simulink library "commcnvintrlv2"  (Simulink 5.0)
libraries: commcnvintrlv2 x4, dspsigattribs x4, commblksprivate x2, commblkintrlv2 x2, simulink x2, dspsigops x1
settings Model: RequirementInfo=9  Creator=mikem  LastModifiedBy=mmclerno  TargetHWChar=2  TargetHWWordLengths=8,16,32,32

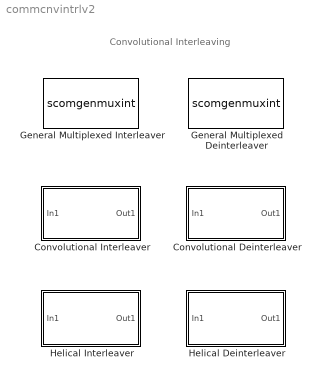
== system commcnvintrlv2 ==
  note: Convolutional Interleaving
  Convolutional Deinterleaver : Subsystem  mask(Convolutional Deinterleaver){N=6, B=2, ic=0}
      mask prompts: N "Rows of shift registers:"; B "Register length step:"; ic "Initial conditions:"
      mask help: A convolutional deinterleaver consists of N shift registers. The ith register has delay (N-i)*B where B is a specified register length step. With each new input symbol, a commutator switches to a new register and the new symbol is shifted in while the oldest symbol in that register is shifted out. When the commutator reaches the Nth register, upon the next new input, it returns to the first register.
      mask Help: helpview(commbhelp)
      mask Display: disp('Convolutional\nDeinterleaver');
  Convolutional Interleaver : Subsystem  mask(Convolutional Interleaver){N=6, B=2, ic=0}
      mask prompts: N "Rows of shift registers:"; B "Register length step:"; ic "Initial conditions:"
      mask help: A convolutional interleaver consists of N shift registers. The ith register has delay (i-1)*B where B is a specified register length step. With each new input symbol, a commutator switches to a new register and the new symbol is shifted in while the oldest symbol in that register is shifted out. When the commutator reaches the Nth register, upon the next new input, it returns to the first register.
      mask Help: helpview(commbhelp)
      mask Display: disp('Convolutional\nInterleaver');
  General Multiplexed Deinterleaver : S-Function  FunctionName=scomgenmuxint  Parameters=delayinverse, real(ic), imag(ic)  mask(General Multiplexed Deinterleaver){delay=[2 0 1 3 10], ic=0}
      mask prompts: delay "Interleaver delay (samples):"; ic "Initial conditions:"
      mask help:
      | A general multiplexed deinterleaver consists of N registers.  With each new input symbol, a commutator switches to a new register and the new symbol is shifted in while the oldest symbol in that register is shifted out.  When the commutator reaches the Nth register, upon the next new input, it returns to the first register.
      |
      | The multiplexed deinterleaver associated with a general multiplexed interleaver has the same number of registers as the interleaver.  The delay in a particular deinterleaver register depends on the largest interleaver delay minus the interleaver delay for the given register.
      mask init:
      | delayinverse=max(delay)-delay;
      mask Help: helpview(commbhelp)
      mask Display: disp('General\nMultiplexed\nDeinterleaver');
  General Multiplexed Interleaver : S-Function  FunctionName=scomgenmuxint  Parameters=delay, real(ic), imag(ic)  mask(General Multiplexed Interleaver){delay=[2 0 1 3 10], ic=0}
      mask prompts: delay "Interleaver delay (samples):"; ic "Initial conditions:"
      mask help: A general multiplexed interleaver consists of N registers, each with a specified delay. With each new input symbol, a commutator switches to a new register and the new symbol is shifted in while the oldest symbol in that register is shifted out. When the commutator reaches the Nth register, upon the next new input, it returns to the first register.
      mask Help: helpview(commbhelp)
      mask Display: disp('General\nMultiplexed\nInterleaver');
  Helical Deinterleaver : Subsystem  mask(Helical Deinterleaver){C=6, N=4, s=1, ic=0}
      mask prompts: C "Number of columns in helical array:"; N "Group size:"; s "Helical array step size:"; ic "Initial condition:"
      mask help:
      | Restore the ordering of symbols input to a matching helical interleaver.  The operation of a helical deinterleaver is defined by a helical array with C columns.  The input to the helical deinterleaver must have width C*N.  Received symbols are entered row-by-row into the helical array.  The block processes the symbols in the helical array in groups of size N and assigns an index k to each group, beginning with k=1 at the start of the simulation.  After a delay, the kth output group is read sequentially down column k mod C of the helical array and beginning in row 1+(k-1)*s, where s is the helical array step size.
      |
      | The helical array step size must be a nonnegative integer and the initial condition must be a scalar.
      mask init:
      | if s<0
      |     error('The helical array step size must be a nonnegative integer.');
      | end
      | 
      | if length(ic)~=1
      |    error('The initial condition must be a scalar.');
      | end
      | 
      | if(C<=0)
      |    error('The number of columns in helical array must be a nonnegative integer.');
      | end
      | 
      | if(N<=0)
      |    error('The group size must be a nonnegative integer.');
      | end
      mask Help: helpview(commbhelp)
      mask Display: disp('Helical\nDeinterleaver');
  Helical Interleaver : Subsystem  mask(Helical Interleaver){C=6, N=4, s=1, ic=0}
      mask prompts: C "Number of columns in helical array:"; N "Group size:"; s "Helical array step size:"; ic "Initial condition:"
      mask help:
      | Permute input vector using a helical array with C columns.  The input to the helical interleaver must have width C*N.  The block processes the input in groups of size N and assigns an index to each group, beginning with k=1 at the start of the simulation.  The kth group of N symbols is entered sequentially down column k mod C of the helical array and beginning in row 1+(k-1)*s, where s is the helical array step size.  The helical interleaver output is then read row-by-row from the helical array.
      |
      | The helical array step size must be a nonnegative integer and the initial condition must be a scalar.
      mask init:
      | if s<0
      |     error('The helical array step size must be a nonnegative integer.');
      | end
      | 
      | if length(ic)~=1
      | error('The initial condition must be a scalar.');
      | end
      | 
      | if(C<=0)
      |    error('The number of columns in helical array must be a nonnegative integer.');
      | end
      | 
      | if(N<=0)
      |    error('The group size must be a nonnegative integer.');
      | end
      mask Help: helpview(commbhelp)
      mask Display: disp('Helical\nInterleaver');

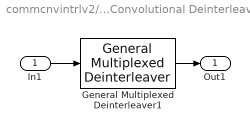
== system commcnvintrlv2/Convolutional Deinterleaver ==
  In1 : Inport
  General Multiplexed Deinterleaver1 : commcnvintrlv2/General Multiplexed Deinterleaver  delay=[0:B:B*(N-1)]'  ic=ic
  Out1 : Outport
  wires:
  In1/1 -> General Multiplexed Deinterleaver1/1
  General Multiplexed Deinterleaver1/1 -> Out1/1

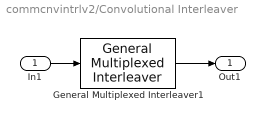
== system commcnvintrlv2/Convolutional Interleaver ==
  In1 : Inport
  General Multiplexed Interleaver1 : commcnvintrlv2/General Multiplexed Interleaver  delay=[0:B:B*(N-1)]'  ic=ic
  Out1 : Outport
  wires:
  In1/1 -> General Multiplexed Interleaver1/1
  General Multiplexed Interleaver1/1 -> Out1/1

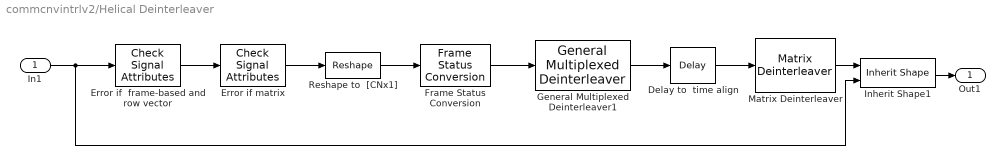
== system commcnvintrlv2/Helical Deinterleaver ==
  In1 : Inport
  Delay to  time align : dspsigops/Delay  dly_unit=Samples  delay=mod(C*N-s*C*(C-1),C*N)  ic_detail=off  dif_ic_for_ch=off  dif_ic_for_dly=off  ic=0  reset_popup=None
  Error if  frame-based and row vector : dspsigattribs/Check Signal Attributes  SigAttribCheckMethod=Matches attributes exactly  Complexity=Ignore  Frame=Frame-based  DimsCheckMethod=Is...  Dimensions=Row vector (2-D)  DatatypeCheckMethod=Ignore  DatatypeGeneral=Boolean  DtypeFloatSpecific=Any floating-point  DtypeFixedSpecific=Any fixed-point  DtypeIntSpecific=Any integer  SampleMode=Ignore
  Error if matrix : dspsigattribs/Check Signal Attributes  SigAttribCheckMethod=Matches attributes exactly  Complexity=Ignore  Frame=Ignore  DimsCheckMethod=Is...  Dimensions=Full matrix (2-D)  DatatypeCheckMethod=Ignore  DatatypeGeneral=Boolean  DtypeFloatSpecific=Any floating-point  DtypeFixedSpecific=Any fixed-point  DtypeIntSpecific=Any integer  SampleMode=Ignore
  Frame Status Conversion : dspsigattribs/Frame Status Conversion  growRefPort=off  outframe=Frame-based
  General Multiplexed Deinterleaver1 : commcnvintrlv2/General Multiplexed Deinterleaver  delay=[0:s:(C-1)*s]'  ic=ic
  Inherit Shape1 : commblksprivate/Inherit Shape
  Matrix Deinterleaver : commblkintrlv2/Matrix Deinterleaver  Nrows=C  Ncols=N
  Reshape to  [CNx1] : simulink/Math Operations/Reshape  OutputDimensionality=Customize  OutputDimensions=[C*N,1]
  Out1 : Outport
  wires:
  Frame Status Conversion/1 -> General Multiplexed Deinterleaver1/1
  General Multiplexed Deinterleaver1/1 -> Delay to  time align/1
  Matrix Deinterleaver/1 -> Inherit Shape1/1
  Inherit Shape1/1 -> Out1/1
  In1/1 -> Inherit Shape1/2, Error if  frame-based and row vector/1
  Reshape to  [CNx1]/1 -> Frame Status Conversion/1
  Error if  frame-based and row vector/1 -> Error if matrix/1
  Error if matrix/1 -> Reshape to  [CNx1]/1
  Delay to  time align/1 -> Matrix Deinterleaver/1

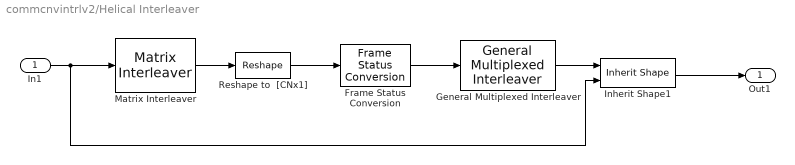
== system commcnvintrlv2/Helical Interleaver ==
  In1 : Inport
  Frame Status Conversion : dspsigattribs/Frame Status Conversion  growRefPort=off  outframe=Frame-based
  General Multiplexed Interleaver : commcnvintrlv2/General Multiplexed Interleaver  delay=[0:s:(C-1)*s]'  ic=ic
  Inherit Shape1 : commblksprivate/Inherit Shape
  Matrix Interleaver : commblkintrlv2/Matrix Interleaver  Nrows=C  Ncols=N
  Reshape to  [CNx1] : simulink/Math Operations/Reshape  OutputDimensionality=Customize  OutputDimensions=[C*N,1]
  Out1 : Outport
  wires:
  In1/1 -> Matrix Interleaver/1, Inherit Shape1/2
  Frame Status Conversion/1 -> General Multiplexed Interleaver/1
  General Multiplexed Interleaver/1 -> Inherit Shape1/1
  Inherit Shape1/1 -> Out1/1
  Matrix Interleaver/1 -> Reshape to  [CNx1]/1
  Reshape to  [CNx1]/1 -> Frame Status Conversion/1
